simulink subsystem "CASE1"  (R2022b)
settings: Solver=VariableStepAuto  StartTime=0.0  StopTime=10.0  RelTol=1e-3
libraries: simulink x1
settings Model: Creator=User  LastModifiedBy=User

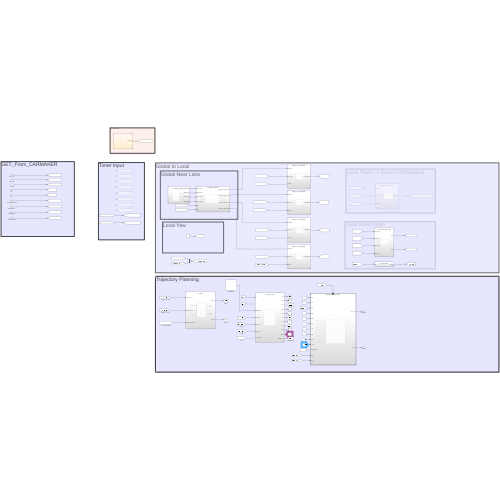
[thumbnail: Simulink's stored preview of the top-level diagram]
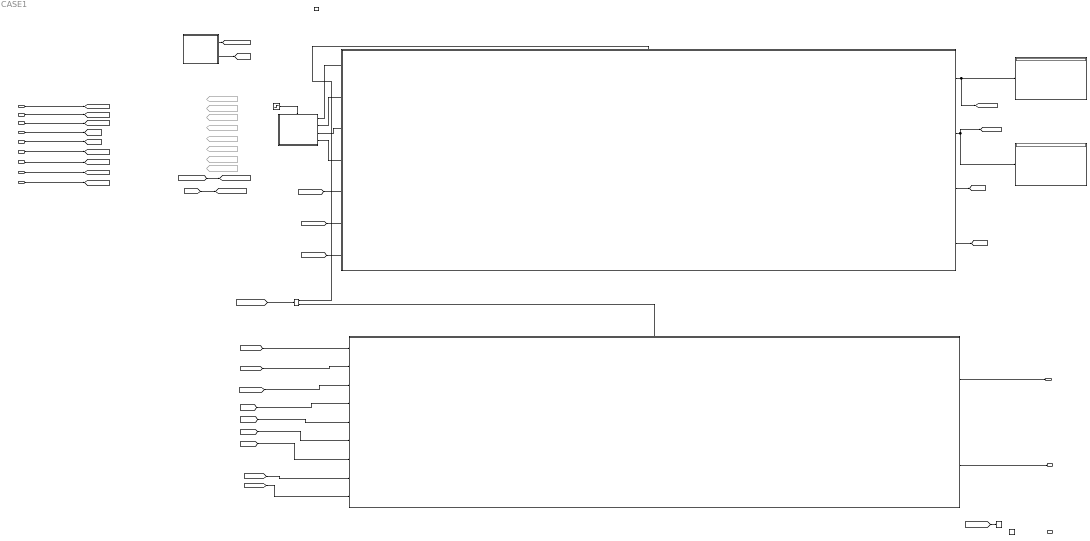
== system CASE1 ==
  note: Timer Input
  note: GET_From_CARMAKER
  note: Do Not Modify !!
  Car_x_pos : Inport
  Car_y_pos : Inport  Port=2
  Car_yaw : Inport  Port=3
  Car_v : Inport  Port=4
  Car_a : Inport  Port=5
  Car_Moved_Distance : Inport  Port=6
  Global_Map_X : Inport  Port=7
  Global_Map_Y : Inport  Port=8
  Global_Traffic_Info : Inport  Port=9
  Trigger : TriggerPort  TriggerType=function-call  VariantControl=(inherit)  PortDimensions=1
  Chart : Stateflow chart  TreatAsAtomicUnit=on
  Compare To Constant : simulink/Logic and Bit Operations/Compare To Constant  relop=>=  const=250  OutDataTypeStr=boolean
  Constant : Constant
  Display1 : Display
  Display2 : Display
  Function-Call Split : FunctionCallSplit  IconShape=distinctive  NumOutputPorts=2  OutputPortLayout=default
  Global to Local : Subsystem
  Goto : Goto  Commented=on  GotoTag=t_10ms
  Goto1 : Goto  Commented=on  GotoTag=t_25ms
  Goto2 : Goto  Commented=on  GotoTag=t_50ms
  Goto3 : Goto  Commented=on  GotoTag=t_100ms
  Goto4 : Goto  Commented=on  GotoTag=t_250ms
  Goto5 : Goto  Commented=on  GotoTag=t_500ms
  Goto6 : Goto  Commented=on  GotoTag=t_1000ms
  Goto7 : Goto  Commented=on  GotoTag=Initial
  Step : Step  Time=0.001
  Subsystem Reference5 : Subsystem  ReferencedSubsystem=Global_Line_Divide
  Trajectory Planning : Subsystem
  Yaw_Value : Outport
  s_d_value : Outport  Port=2
  Out1 : Outport  Port=3
  wires:
  Chart/2(do_Logic_2()) -> [do_logic2]
  Chart/1(do_Logic_1()) -> [do_Logic]
  [do_Logic] -> [t_100ms]
  Global_Traffic_Info/1 -> [global_traffic_info]
  Global_Map_Y/1 -> [global_mapy]
  Car_v/1 -> [v_ego_car]
  Global_Map_X/1 -> [global_mapx]
  Car_y_pos/1 -> [global_ego_car_y]
  Car_yaw/1 -> [global_car_yaw]
  Car_x_pos/1 -> [global_ego_car_x]
  Car_Moved_Distance/1 -> [car_moved_distance]
  Car_a/1 -> [a_ego_car]
  [do_logic2] -> [t_50ms]
  Step/1 -> Subsystem Reference5/Trigger
  Trajectory Planning/1(Yaw_Value) -> Yaw_Value/1
  Trajectory Planning/2(s_d_value) -> s_d_value/1
  [local_mapx] -> Trajectory Planning/8(local_map_Y2)
  [local_mapy] -> Trajectory Planning/9(local_map_Y3)
  [a_ego_car] -> Trajectory Planning/7(local_map_X2)
  [v_ego_car] -> Trajectory Planning/6(v_ego_car)
  [yaw_local] -> Trajectory Planning/5(local_map_Y1)
  [yaw_road] -> Trajectory Planning/4(local_map_X1)
  [car_moved_distance] -> Trajectory Planning/3(In3)
  [local_mapx] -> Trajectory Planning/1(local_map_X)
  [local_mapy] -> Trajectory Planning/2(local_map_Y)
  Subsystem Reference5/1 -> Global to Local/1(Global_Lane1)
  Subsystem Reference5/2 -> Global to Local/2(Global_Lane2)
  Subsystem Reference5/3 -> Global to Local/3(Global_Lane3)
  Subsystem Reference5/4 -> Global to Local/4(Global_Lane4)
  [global_ego_car_x] -> Global to Local/5(ego_x)
  [global_ego_car_y] -> Global to Local/6(ego_y)
  Global to Local/1(mapx) -> Display1/1, [local_mapx]
  Global to Local/2(mapx1) -> Display2/1, [local_mapy]
  Global to Local/3(yaw_road) -> [yaw_road]
  Global to Local/4(y_local) -> [yaw_local]
  [global_car_yaw] -> Global to Local/7(In1)
  [t_100ms] -> Function-Call Split/1
  Function-Call Split/1 -> Global to Local/Trigger
  Function-Call Split/2 -> Trajectory Planning/Trigger
  [car_moved_distance] -> Compare To Constant/1

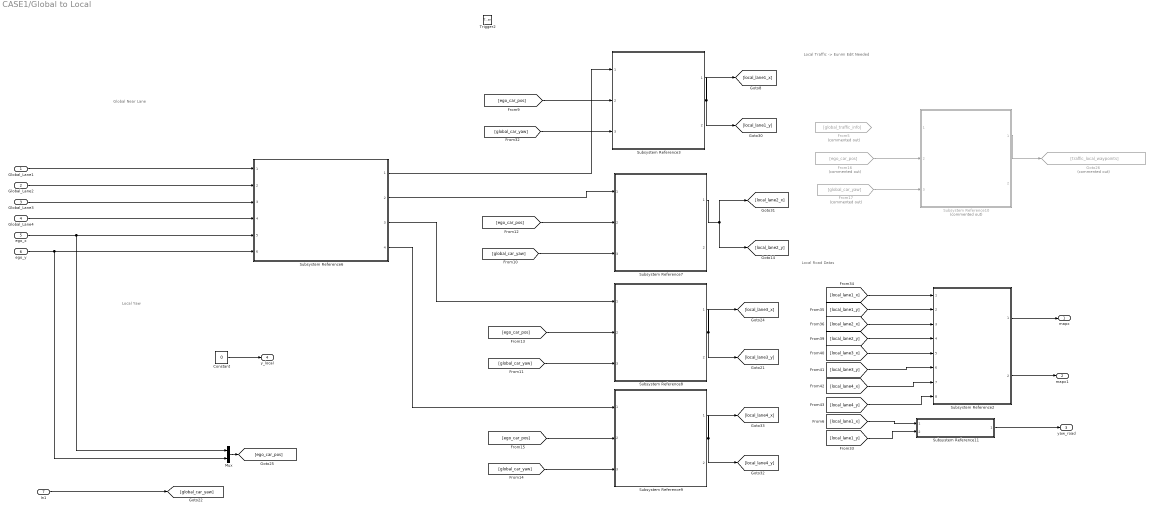
== system CASE1/Global to Local ==
  note: Global Near Lane
  note: Local Traffic -> Eunmi Edit Needed
  note: Local Yaw
  note: Local Road Datas
  Global_Lane1 : Inport
  Global_Lane2 : Inport  Port=2
  Global_Lane3 : Inport  Port=3
  Global_Lane4 : Inport  Port=4
  ego_x : Inport  Port=5
  ego_y : Inport  Port=6
  In1 : Inport  Port=7
  Trigger2 : TriggerPort  TriggerType=function-call  VariantControl=(inherit)  PortDimensions=1
  Constant : Constant  Value=0
  From16 : From  Commented=on  GotoTag=ego_car_pos
  From17 : From  Commented=on  GotoTag=global_car_yaw
  From5 : From  Commented=on  GotoTag=global_traffic_info
  Goto26 : Goto  Commented=on  GotoTag=traffic_local_waypoints
  Mux : Mux  Inputs=2
  Subsystem Reference10 : Subsystem  Commented=on  ReferencedSubsystem=Global_to_Local_WayPoints
  Subsystem Reference11 : Subsystem  ReferencedSubsystem=Get_Yaw_Road
  Subsystem Reference2 : Subsystem  ReferencedSubsystem=Get_Lanes_and_Return_Map
  Subsystem Reference{3,7..9} (4 alike) : Subsystem  ReferencedSubsystem=Global_to_Local_WayPoints
  Subsystem Reference6 : Subsystem  ReferencedSubsystem=Global_Near_Waypoints
  mapx : Outport
  mapx1 : Outport  Port=2
  yaw_road : Outport  Port=3
  y_local : Outport  Port=4
  wires:
  In1/1 -> [global_car_yaw]
  Global_Lane4/1 -> Subsystem Reference6/4
  Global_Lane1/1 -> Subsystem Reference6/1
  Global_Lane3/1 -> Subsystem Reference6/3
  Global_Lane2/1 -> Subsystem Reference6/2
  [ego_car_pos] -> Subsystem Reference3/2
  [global_car_yaw] -> Subsystem Reference7/3
  Subsystem Reference6/4 -> Subsystem Reference9/1
  ego_x/1 -> Subsystem Reference6/5, Mux/1
  From16/1 -> Subsystem Reference10/2
  [ego_car_pos] -> Subsystem Reference9/2
  [ego_car_pos] -> Subsystem Reference7/2
  [ego_car_pos] -> Subsystem Reference8/2
  [local_lane4_y] -> Subsystem Reference2/8
  From17/1 -> Subsystem Reference10/3
  [local_lane1_x] -> Subsystem Reference2/1
  Subsystem Reference6/1 -> Subsystem Reference3/1
  Mux/1 -> [ego_car_pos]
  Constant/1 -> y_local/1
  [local_lane4_x] -> Subsystem Reference2/7
  Subsystem Reference3/1 -> [local_lane1_y], [local_lane1_x]
  Subsystem Reference2/2 -> mapx1/1
  Subsystem Reference9/1 -> [local_lane4_y], [local_lane4_x]
  Subsystem Reference6/2 -> Subsystem Reference7/1
  Subsystem Reference6/3 -> Subsystem Reference8/1
  ego_y/1 -> Subsystem Reference6/6, Mux/2
  [local_lane2_y] -> Subsystem Reference2/4
  [local_lane1_y] -> Subsystem Reference2/2
  [global_car_yaw] -> Subsystem Reference9/3
  [global_car_yaw] -> Subsystem Reference3/3
  [local_lane2_x] -> Subsystem Reference2/3
  Subsystem Reference11/1 -> yaw_road/1
  Subsystem Reference10/1 -> Goto26/1
  [global_car_yaw] -> Subsystem Reference8/3
  Subsystem Reference2/1 -> mapx/1
  Subsystem Reference7/1 -> [local_lane2_x], [local_lane2_y]
  [local_lane3_x] -> Subsystem Reference2/5
  [local_lane1_x] -> Subsystem Reference11/1
  [local_lane1_y] -> Subsystem Reference11/2
  [local_lane3_y] -> Subsystem Reference2/6
  Subsystem Reference8/1 -> [local_lane3_y], [local_lane3_x]

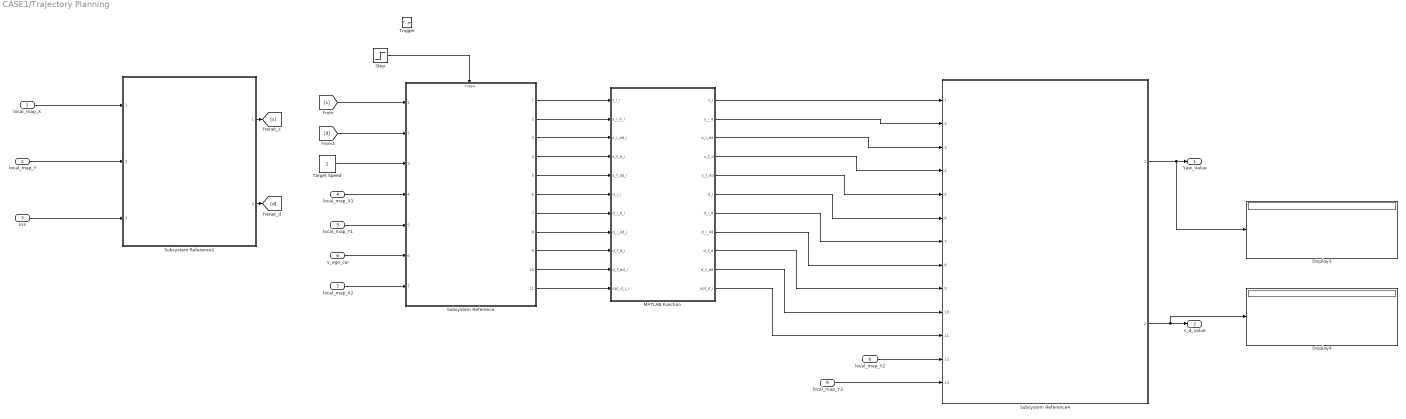
== system CASE1/Trajectory Planning ==
  local_map_X : Inport
  local_map_Y : Inport  Port=2
  In3 : Inport  Port=3
  local_map_X1 : Inport  Port=4
  local_map_Y1 : Inport  Port=5
  v_ego_car : Inport  Port=6
  local_map_X2 : Inport  Port=7
  local_map_Y2 : Inport  Port=8
  local_map_Y3 : Inport  Port=9
  Trigger : TriggerPort  TriggerType=function-call  VariantControl=(inherit)  PortDimensions=1
  Display3 : Display
  Display4 : Display
  MATLAB Function : MATLAB Function  TreatAsAtomicUnit=on
  Step : Step  Time=0.1
  Subsystem Reference : Subsystem  ReferencedSubsystem=Init_Frenet_Value
  Subsystem Reference1 : Subsystem  ReferencedSubsystem=Get_Frenet
  Subsystem Reference4 : Subsystem  ReferencedSubsystem=Calculate_Frenet_and_Paths
  Target Speed : Constant
  Yaw_Value : Outport
  s_d_value : Outport  Port=2
  wires:
  Subsystem Reference/11 -> MATLAB Function/11(opt_d_i_i)
  Subsystem Reference/10 -> MATLAB Function/10(d_f_dd_i)
  Subsystem Reference/9 -> MATLAB Function/9(d_f_d_i)
  Subsystem Reference/8 -> MATLAB Function/8(d_i_dd_i)
  Subsystem Reference/7 -> MATLAB Function/7(d_i_d_i)
  Subsystem Reference/6 -> MATLAB Function/6(d_i_i)
  Subsystem Reference/5 -> MATLAB Function/5(s_f_dd_i)
  Subsystem Reference/3 -> MATLAB Function/3(s_i_dd_i)
  Subsystem Reference/2 -> MATLAB Function/2(s_i_d_i)
  Step/1 -> Subsystem Reference/Trigger
  local_map_Y3/1 -> Subsystem Reference4/13
  local_map_Y2/1 -> Subsystem Reference4/12
  local_map_X2/1 -> Subsystem Reference/7
  v_ego_car/1 -> Subsystem Reference/6
  local_map_Y1/1 -> Subsystem Reference/5
  local_map_X1/1 -> Subsystem Reference/4
  In3/1 -> Subsystem Reference1/3
  local_map_Y/1 -> Subsystem Reference1/2
  local_map_X/1 -> Subsystem Reference1/1
  MATLAB Function/10(d_f_dd) -> Subsystem Reference4/10
  Subsystem Reference/1 -> MATLAB Function/1(s_i_i)
  MATLAB Function/2(s_i_d) -> Subsystem Reference4/2
  [s] -> Subsystem Reference/1
  Subsystem Reference4/2 -> s_d_value/1, Display4/1
  MATLAB Function/3(s_i_dd) -> Subsystem Reference4/3
  Subsystem Reference4/1 -> Yaw_Value/1, Display3/1
  Subsystem Reference1/2 -> [d]
  Subsystem Reference1/1 -> [s]
  MATLAB Function/5(s_f_dd) -> Subsystem Reference4/5
  MATLAB Function/8(d_i_dd) -> Subsystem Reference4/8
  MATLAB Function/6(d_i) -> Subsystem Reference4/6
  MATLAB Function/11(opt_d_i) -> Subsystem Reference4/11
  Target Speed/1 -> Subsystem Reference/3
  MATLAB Function/1(s_i) -> Subsystem Reference4/1
  [d] -> Subsystem Reference/2
  MATLAB Function/9(d_f_d) -> Subsystem Reference4/9
  MATLAB Function/7(d_i_d) -> Subsystem Reference4/7
  Subsystem Reference/4 -> MATLAB Function/4(s_f_d_i)
  MATLAB Function/4(s_f_d) -> Subsystem Reference4/4

== matlab function CASE1/Trajectory Planning/MATLAB Function ==
  data: s_i_i input; s_i output; s_i_d_i input; s_i_dd_i input; s_f_d_i input; s_f_dd_i input; d_i_i input; d_i_d_i input; d_i_dd_i input; d_f_d_i input; d_f_dd_i input; opt_d_i_i input; s_i_d output; s_i_dd output; s_f_d output; s_f_dd output; d_i output; d_i_d output; d_i_dd output; d_f_d output; d_f_dd output; opt_d_i output
function [s_i,s_i_d,s_i_dd,s_f_d,s_f_dd,d_i,d_i_d,d_i_dd,d_f_d,d_f_dd,opt_d_i] = fcn(s_i_i,s_i_d_i,s_i_dd_i,s_f_d_i,s_f_dd_i,d_i_i,d_i_d_i,d_i_dd_i,d_f_d_i,d_f_dd_i,opt_d_i_i)

    persistent s1 s2 s3 s4 s5 d1 d2 d3 d4 d5 o1
    
    % lane_road_value가 비어있으면 처음으로 값을 대입
    if isempty(s1)
        s1 = s_i_i; % 예시: 글로벌 차선 초기 값 line 입력
        s2 = s_i_d_i;
        s3 = s_i_dd_i;
        s4 = s_f_d_i;
        s5 = s_f_dd_i;
        d1 = d_i_i; % 예시: 글로벌 차선 초기 값 line 입력
        d2 = d_i_d_i;
        d3 = d_i_dd_i;
        d4 = d_f_d_i;
        d5 = d_f_dd_i;
        o1 = opt_d_i_i;
    end
    
    s_i =s1;
    s_i_d =s2; 
    s_i_dd =s3; 
    s_f_d =s4;
    s_f_dd =s5;
    d_i = d1;
    d_i_d = d2;
    d_i_dd = d3;
    d_f_d = d4;
    d_f_dd = d5;
    opt_d_i = o1;

end

== stateflow chart CASE1/Chart ==
  (default) -> (junction 1)
  (junction 1) -> (junction 3) [order 1] : [i<199]
      | {i = i + 1;}
  (junction 1) -> (junction 7) [order 2] : {i=0;}
  (junction 3) -> (junction 5)
  (junction 5) -> (junction 7)
  (junction 7) -> (junction 10)
  (junction 10) -> (junction 12) [order 1] : [mod(i,100)==0]
      | {do_Logic_1;}
  (junction 10) -> (junction 18) [order 2]
  (junction 12) -> (junction 16)
  (junction 16) -> (junction 18)
  (junction 18) -> (junction 36)
  (junction 36) -> (junction 35) [order 1] : [mod(i,50)==0]
      | {do_Logic_2;}
  (junction 36) -> (junction 34) [order 2]
  (junction 35) -> (junction 32)
  (junction 32) -> (junction 34)
  (junction 34) -> (junction 39)
  data: i local =0
  events: do_Logic_1 output FUNCTION_CALL_EVENT; do_Logic_2 output FUNCTION_CALL_EVENT
